simulink model "ServoBD"  (R2018a)
settings: Solver=VariableStepAuto  StartTime=0.0  StopTime=10.0  RelTol=1e-3  EnableMultiTasking=on
settings Model: Creator=retro  LastModifiedBy=HOME
settings OptimizationCC: LifeSpan=inf
settings DebuggingCC: SFUnexpectedBacktrackingDiag=warning  SFNoUnconditionalDefaultTransitionDiag=warning  SFExecutionAtInitializationDiag=none
settings CodeAppCC: StateflowObjectComments=on
settings GRTTargetCC: TargetLangStandard=C89/C90 (ANSI)  GeneratePreprocessorConditionals=Disable all
settings ConfigComp: CovMetricSettings=dw  CovHtmlReporting=on  CovSaveCumulativeToWorkspaceVar=on  CovSaveSingleToWorkspaceVar=on  CovExternalEMLEnable=off

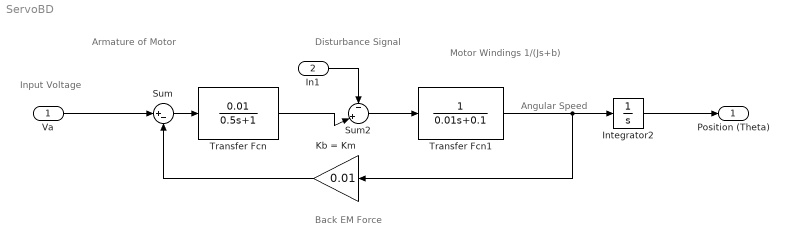
== system ServoBD ==
  note: Back
      | EM Force
  note: Angular
      | Speed
  note: Motor Windings
      | 1/(Js+b)
  note: Disturbance Signal
  note: Armature of Motor
  note: Input Voltage
  Va : Inport
  In1 : Inport  Port=2
  Integrator2 : Integrator
  Kb = Km : Gain  Gain=0.01
  Sum : Sum  Inputs=|+-
  Sum2 : Sum  Inputs=-|+|
  Transfer Fcn : TransferFcn  Numerator=[0.01]  Denominator=[0.5 1]
  Transfer Fcn1 : TransferFcn  Denominator=[0.01 0.1]
  Position (Theta) : Outport
  wires:
  Va/1 -> Sum/1
  Integrator2/1 -> Position (Theta)/1
  Sum/1 -> Transfer Fcn/1
  Transfer Fcn/1 -> Sum2/2
  In1/1 -> Sum2/1
  Sum2/1 -> Transfer Fcn1/1
  Transfer Fcn1/1 -> Integrator2/1, Kb = Km/1
  Kb = Km/1 -> Sum/2
